simulink model "main_sim_sl"  (R2023b)
settings: Solver=VariableStepAuto  StartTime=0.0  StopTime=10.0  RelTol=1e-3
undefined symbols (not defined in the file or in its folder): sim_msg
settings Model: Creator=tard  LastModifiedBy=tard

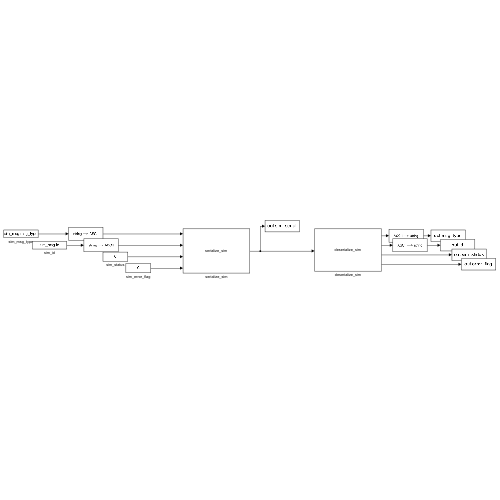
[thumbnail: Simulink's stored preview of the top-level diagram]
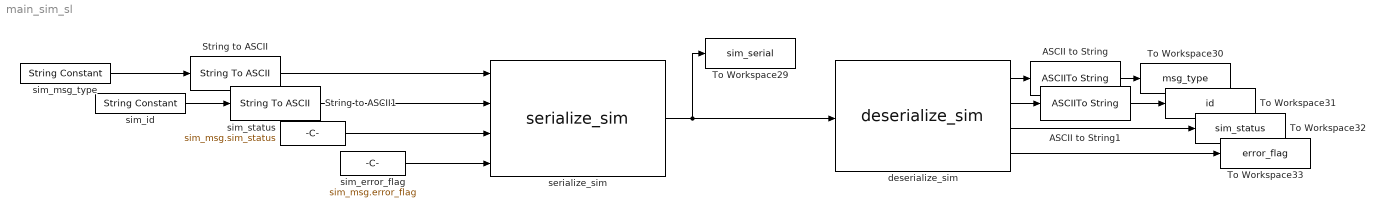
== system main_sim_sl ==
  ASCII to String : ASCIIToString
  ASCII to String1 : ASCIIToString
  String to ASCII : StringToASCII
  String to ASCII1 : StringToASCII
  To Workspace29 : ToWorkspace  VariableName=sim_serial  SaveFormat=Timeseries  SampleTime=-1
  To Workspace30 : ToWorkspace  VariableName=msg_type  SaveFormat=Timeseries  SampleTime=-1
  To Workspace31 : ToWorkspace  VariableName=id  SaveFormat=Timeseries  SampleTime=-1
  To Workspace32 : ToWorkspace  VariableName=sim_status  SaveFormat=Timeseries  SampleTime=-1
  To Workspace33 : ToWorkspace  VariableName=error_flag  SaveFormat=Timeseries  SampleTime=-1
  deserialize_sim : S-Function  FunctionName=deserialize_sim  SFunctionDeploymentMode=off  EnableBusSupport=off
  serialize_sim : S-Function  FunctionName=serialize_sim  SFunctionDeploymentMode=off  EnableBusSupport=off
  sim_error_flag : Constant  Value=sim_msg.error_flag
  sim_id : StringConstant  String=sim_msg.id
  sim_msg_type : StringConstant  String=sim_msg.msg_type
  sim_status : Constant  Value=sim_msg.sim_status
  wires:
  sim_status/1 -> serialize_sim/3
  sim_id/1 -> String to ASCII1/1
  sim_msg_type/1 -> String to ASCII/1
  deserialize_sim/3 -> To Workspace32/1
  deserialize_sim/2 -> ASCII to String1/1
  deserialize_sim/1 -> ASCII to String/1
  sim_error_flag/1 -> serialize_sim/4
  serialize_sim/1 -> To Workspace29/1, deserialize_sim/1
  deserialize_sim/4 -> To Workspace33/1
  String to ASCII/1 -> serialize_sim/1
  String to ASCII1/1 -> serialize_sim/2
  ASCII to String/1 -> To Workspace30/1
  ASCII to String1/1 -> To Workspace31/1
